simulink model "example"  (Simulink 8.5)
settings: Solver=ode15s  StartTime=0.0  StopTime=8*24*3600  RelTol=1e-3
undefined symbols (not defined in the file or in its folder): B, U, x0
settings Model: Creator=M.Sparnaaij  LastModifiedBy=Martijn  ExtModeTrigMode=oneshot  ExtModeArmWhenConnect=off
settings DataIOCC: LimitDataPoints=off  SignalLoggingName=sigsOut
settings OptimizationCC: BooleanDataType=off
settings DebuggingCC: SaveWithParameterizedLinksMsg=none  SignalResolutionControl=TryResolveAllWithWarning  MultiTaskDSMMsg=warning  MultiTaskCondExecSysMsg=none  FcnCallInpInsideContextMsg=EnableAllAsWarning  StrictBusMsg=None
settings HardwareCC: TargetUnknown=on

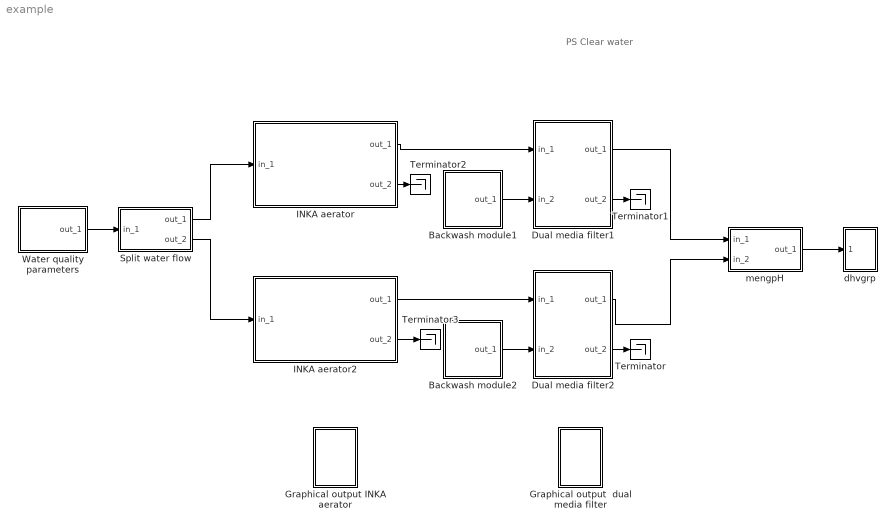
== system example ==
  note: PS Clear water
  Backwash module1 : Subsystem  Description=During a simulation the filter can be backwashed with the backwash module, so a number of successive filterruns can be simulated.
      mask init:
      | filenaam='./StimelaData/Backwash module1.mat';
      | 
      | [Pn,Fn,Fext]=Fileprop(filenaam);
      | 
      | errstr = st_UniqName(filenaam,'filenaam=''','SubSystem','OpenFcn');
      | if errstr, error([errstr 'The filename "' filenaam '" is already in use. Choose a different filename.']), end
      | 
      | P = bacwa1_p(filenaam);
      | [B,x0,U]=bacwa1_i(filenaam);
      settings: OpenFcn=|
      | filenaam='./StimelaData/Backwash module1.mat';
      | st_ParameterInput('init',gcb,filenaam,'bacwa1');
      mask Display:
      | plot(0,0,100,100,[80,80,20,20],[80,20,20,80],[40,42,38,40,40],[70,67,67,70,30],[60,62,58,60,60],[70,67,67,70,30]);
      | disp('')
      | text(50,50,'bacwa1', 'horizontalAlignment', 'center', 'verticalAlignment', 'middle');
      | text(50,0,Fn, 'horizontalAlignment', 'center', 'verticalAlignment', 'base');
  Backwash module2 : Subsystem  Description=During a simulation the filter can be backwashed with the backwash module, so a number of successive filterruns can be simulated.
      mask init:
      | filenaam='./StimelaData/Backwash module2.mat';
      | 
      | [Pn,Fn,Fext]=Fileprop(filenaam);
      | 
      | errstr = st_UniqName(filenaam,'filenaam=''','SubSystem','OpenFcn');
      | if errstr, error([errstr 'The filename "' filenaam '" is already in use. Choose a different filename.']), end
      | 
      | P = bacwa1_p(filenaam);
      | [B,x0,U]=bacwa1_i(filenaam);
      settings: OpenFcn=|
      | filenaam='./StimelaData/Backwash module2.mat';
      | st_ParameterInput('init',gcb,filenaam,'bacwa1');
      mask Display:
      | plot(0,0,100,100,[80,80,20,20],[80,20,20,80],[40,42,38,40,40],[70,67,67,70,30],[60,62,58,60,60],[70,67,67,70,30]);
      | disp('')
      | text(50,50,'bacwa1', 'horizontalAlignment', 'center', 'verticalAlignment', 'middle');
      | text(50,0,Fn, 'horizontalAlignment', 'center', 'verticalAlignment', 'base');
  Dual media filter1 : Subsystem  Description=This model calculates the removal of suspended solids with a dual media filter.
      mask init:
      | filenaam='./StimelaData/Dual_media_filter1.mat';
      | 
      | [Pn,Fn,Fext]=Fileprop(filenaam);
      | 
      | errstr = st_UniqName(filenaam,'filenaam=''','SubSystem','OpenFcn');
      | if errstr, error([errstr 'The filename "' filenaam '" is already in use. Choose a different filename.']), end
      | 
      | P = dubfil_p(filenaam);
      | [B,x0,U]=dubfil_i(filenaam);
      settings: OpenFcn=|
      | filenaam='./StimelaData/Dual_media_filter1.mat';
      | st_ParameterInput('init',gcb,filenaam,'dubfil');
      mask Display:
      | plot(0,0,100,100,[25.000000,25.000000,75.000000,75.000000,87.500000],[75.000000,25.000000,25.000000,30.000000,30.000000],[87.500000,75.000000,75.000000],[37.500000,37.500000,75.000000],[25.000000,75.000000],[65.000000,65.000000],[25.000000,75.000000],[42.500000,42.500000],[37.500000,42.500000],[52.500000,52.500000],[50.000000,55.000000],[52.500000,52.500000],[62.500000,67.500000],[52.500000,52.500000])
      | disp('')
      | text(50,50,'dubfil', 'horizontalAlignment', 'center', 'verticalAlignment', 'middle');
      | text(50,0,Fn, 'horizontalAlignment', 'center', 'verticalAlignment', 'base');
  Dual media filter2 : Subsystem  Description=This model calculates the removal of suspended solids with a dual media filter.
      mask init:
      | filenaam='./StimelaData/Dual_media_filter2.mat';
      | 
      | [Pn,Fn,Fext]=Fileprop(filenaam);
      | 
      | errstr = st_UniqName(filenaam,'filenaam=''','SubSystem','OpenFcn');
      | if errstr, error([errstr 'The filename "' filenaam '" is already in use. Choose a different filename.']), end
      | 
      | P = dubfil_p(filenaam);
      | [B,x0,U]=dubfil_i(filenaam);
      settings: OpenFcn=|
      | filenaam='./StimelaData/Dual_media_filter2.mat';
      | st_ParameterInput('init',gcb,filenaam,'dubfil');
      mask Display:
      | plot(0,0,100,100,[25.000000,25.000000,75.000000,75.000000,87.500000],[75.000000,25.000000,25.000000,30.000000,30.000000],[87.500000,75.000000,75.000000],[37.500000,37.500000,75.000000],[25.000000,75.000000],[65.000000,65.000000],[25.000000,75.000000],[42.500000,42.500000],[37.500000,42.500000],[52.500000,52.500000],[50.000000,55.000000],[52.500000,52.500000],[62.500000,67.500000],[52.500000,52.500000])
      | disp('')
      | text(50,50,'dubfil', 'horizontalAlignment', 'center', 'verticalAlignment', 'middle');
      | text(50,0,Fn, 'horizontalAlignment', 'center', 'verticalAlignment', 'base');
  Graphical output  dual media filter : Subsystem
      settings: OpenFcn=dubfil_g
      mask Display:
      | plot(0,0,100,100,[80,20,20],[20,20,80],[80,69,60,52,45,39,33,28,24,20],[65,65,64,61,57,52,45,37,30,20])
      | disp('');
      | text(100,100,'dubfil', 'horizontalAlignment', 'right', 'verticalAlignment', 'top');
  Graphical output INKA aerator : Subsystem
      settings: OpenFcn=plaatb_g
      mask Display:
      | plot(0,0,100,100,[80,20,20],[20,20,80],[80,69,60,52,45,39,33,28,24,20],[65,65,64,61,57,52,45,37,30,20])
      | disp('');
      | text(100,100,'plaatb', 'horizontalAlignment', 'right', 'verticalAlignment', 'top');
  INKA aerator : Subsystem  Description=This model calculates the aeration and degassifying with an INKA aerator. The influent carbon dioxide concentration is calculated on the basis of the bicarbonate concentration, the pH, the EGV and the water temperature, so these parameters must always be filled out in the 'Water quality parameters' block.
      mask init:
      | filenaam='./StimelaData/INKA_aerator1.mat';
      | 
      | [Pn,Fn,Fext]=Fileprop(filenaam);
      | 
      | errstr = st_UniqName(filenaam,'filenaam=''','SubSystem','OpenFcn');
      | if errstr, error([errstr 'The filename "' filenaam '" is already in use. Choose a different filename.']), end
      | 
      | P = plaatb_p(filenaam);
      | [B,x0,U]=plaatb_i(filenaam);
      settings: OpenFcn=|
      | filenaam='./StimelaData/INKA_aerator1.mat';
      | st_ParameterInput('init',gcb,filenaam,'plaatb');
      mask Display:
      | plot(0,0,100,100,[20,80,80,20,20],[70,70,20,20,70],[80,90,90,90,9,9,20],[20,20,30,40,40,60,60],[80,20],[50,50],[11,10,8,6],[60,65,68,70],[15,14,12,10,6],[60,64,67,69,70],[78,78],[40,50],[84,83,82,80],[40,45,48,50],[87,86,84,80],[40,45,48,50],[64,64,67,67],[80,77,77,70],[64,73,73,70,70],[80,80,77,77,70],[70,67],[77,77])
      | disp('')
      | text(50,50,'plaatb', 'horizontalAlignment', 'center', 'verticalAlignment', 'middle');
      | text(50,0,Fn, 'horizontalAlignment', 'center', 'verticalAlignment', 'base');
  INKA aerator2 : Subsystem  Description=This model calculates the aeration and degassifying with an INKA aerator. The influent carbon dioxide concentration is calculated on the basis of the bicarbonate concentration, the pH, the EGV and the water temperature, so these parameters must always be filled out in the 'Water quality parameters' block.
      mask init:
      | filenaam='./StimelaData/INKA_aerator2.mat';
      | 
      | [Pn,Fn,Fext]=Fileprop(filenaam);
      | 
      | errstr = st_UniqName(filenaam,'filenaam=''','SubSystem','OpenFcn');
      | if errstr, error([errstr 'The filename "' filenaam '" is already in use. Choose a different filename.']), end
      | 
      | P = plaatb_p(filenaam);
      | [B,x0,U]=plaatb_i(filenaam);
      settings: OpenFcn=|
      | filenaam='./StimelaData/INKA_aerator2.mat';
      | st_ParameterInput('init',gcb,filenaam,'plaatb');
      mask Display:
      | plot(0,0,100,100,[20,80,80,20,20],[70,70,20,20,70],[80,90,90,90,9,9,20],[20,20,30,40,40,60,60],[80,20],[50,50],[11,10,8,6],[60,65,68,70],[15,14,12,10,6],[60,64,67,69,70],[78,78],[40,50],[84,83,82,80],[40,45,48,50],[87,86,84,80],[40,45,48,50],[64,64,67,67],[80,77,77,70],[64,73,73,70,70],[80,80,77,77,70],[70,67],[77,77])
      | disp('')
      | text(50,50,'plaatb', 'horizontalAlignment', 'center', 'verticalAlignment', 'middle');
      | text(50,0,Fn, 'horizontalAlignment', 'center', 'verticalAlignment', 'base');
  Split water flow : Subsystem  Description=splits
      mask init:
      | filenaam='./StimelaData/splits_p.mat';
      | 
      | [Pn,Fn,Fext]=Fileprop(filenaam);
      | 
      | errstr = st_UniqName(filenaam,'filenaam=''','SubSystem','OpenFcn');
      | if errstr, error([errstr 'The filename "' filenaam '" is already in use. Choose a different filename.']), end
      | 
      | P = splits_p(filenaam);
      | [B,x0,U]=splits_i(filenaam);
      settings: OpenFcn=|
      | filenaam='./StimelaData/splits_p.mat';
      | st_ParameterInput('init',gcb,filenaam,'splits');
      mask Display:
      | plot(0,0,100,100,[0 20],[50 50],[0 20],[55 55],[80 100],[80 80],[80 100],[85 85],[80 100],[ 20 20],[80 100],[ 15 15],[20 80 80 20 20],[10 10 90  90 10]);
      | disp('')
      | text(50,50,'splits', 'horizontalAlignment', 'center', 'verticalAlignment', 'middle');
      | text(50,0,Fn, 'horizontalAlignment', 'center', 'verticalAlignment', 'base');
  Terminator{,1..3} (4 alike) : Terminator
  Water quality parameters : Subsystem  Description=The water flow and the water quality data must be filled out in the 'Water quality parameters' block. Each project must start with a 'Water quality parameters' block.
      mask init:
      | filenaam='./StimelaData/Water_qual_param.mat';
      | 
      | [Pn,Fn,Fext]=Fileprop(filenaam);
      | 
      | errstr = st_UniqName(filenaam,'filenaam=''','SubSystem','OpenFcn');
      | if errstr, error([errstr 'The filename "' filenaam '" is already in use. Choose a different filename.']), end
      | 
      | P = invruw_p(filenaam);
      | [B,x0,U]=invruw_i(filenaam);
      settings: OpenFcn=|
      | filenaam='./StimelaData/Water_qual_param.mat';
      | st_ParameterInput('init',gcb,filenaam,'invruw');
      mask Display:
      | plot(0,0,100,100,[80 100],[ 50 50],[80 100],[ 55 55],[20 80 80 20 20],[10 10 90  90 10]);
      | disp('')
      | text(50,50,'invruw', 'horizontalAlignment', 'center', 'verticalAlignment', 'middle');
      | text(50,0,Fn, 'horizontalAlignment', 'center', 'verticalAlignment', 'base');
  dhvgrp : Subsystem  Description=dhvgrp
      mask init:
      | filenaam='./StimelaData/OnLineGraph.mat';
      | 
      | [Pn,Fn,Fext]=Fileprop(filenaam);
      | 
      | errstr = st_UniqName(filenaam,'filenaam=''','SubSystem','OpenFcn');
      | if errstr, error([errstr 'The filename "' filenaam '" is already in use. Choose a different filename.']), end
      | 
      | P = dhvgrp_p(filenaam);
      | [B,x0,U]=dhvgrp_i(filenaam);
      settings: OpenFcn=|
      | filenaam='./StimelaData/OnLineGraph.mat';
      | st_ParameterInput('init',gcb,filenaam,'dhvgrp');
      mask Display:
      | plot(0,0,100,100,[90,10,10,10,90,90,10],[65,65,90,40,40,90,90],[90,78,69,54,40,31,25,10],[77,60,48,46,56,75,81,84])
      | disp('')
  mengpH : Subsystem  Description=mengpH
      mask init:
      | filenaam='./StimelaData/mengpH_p.mat';
      | 
      | [Pn,Fn,Fext]=Fileprop(filenaam);
      | 
      | errstr = st_UniqName(filenaam,'filenaam=''','SubSystem','OpenFcn');
      | if errstr, error([errstr 'The filename "' filenaam '" is already in use. Choose a different filename.']), end
      | 
      | P = mengpH_p(filenaam);
      | [B,x0,U]=mengpH_i(filenaam);
      | V = st_Varia;
      settings: OpenFcn=|
      | filenaam='./StimelaData/mengpH_p.mat';
      | st_ParameterInput('init',gcb,filenaam,'mengpH');
      mask Display:
      | plot(0,0,100,100,[0 20],[85 85],[0 20],[80 80],[0 20],[20 20],[0 20],[15 15],[80 100],[ 50 50],[80 100],[ 55 55],[20 80 80 20 20],[10 10 90  90 10]);
      | disp('')
      | text(50,50,'mengpH', 'horizontalAlignment', 'center', 'verticalAlignment', 'middle');
      | text(50,0,Fn, 'horizontalAlignment', 'center', 'verticalAlignment', 'base');
  wires:
  Split water flow/2(out_2) -> INKA aerator2/1(in_1)
  Split water flow/1(out_1) -> INKA aerator/1(in_1)
  Water quality parameters/1(out_1) -> Split water flow/1(in_1)
  INKA aerator/1(out_1) -> Dual media filter1/1(in_1)
  INKA aerator2/1(out_1) -> Dual media filter2/1(in_1)
  Dual media filter1/1(out_1) -> mengpH/1(in_1)
  Dual media filter2/1(out_1) -> mengpH/2(in_2)
  Backwash module2/1(out_1) -> Dual media filter2/2(in_2)
  Dual media filter2/2(out_2) -> Terminator/1
  Dual media filter1/2(out_2) -> Terminator1/1
  INKA aerator/2(out_2) -> Terminator2/1
  INKA aerator2/2(out_2) -> Terminator3/1
  Backwash module1/1(out_1) -> Dual media filter1/2(in_2)
  mengpH/1(out_1) -> dhvgrp/1(in_1)

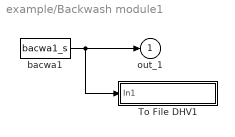
== system example/Backwash module1 ==
  To File DHV1 : Subsystem  mask(To File DHV){naam=[filenaam(1:length(filenaam)-4) '_out.sti']}
      mask prompts: naam "Naam van bestand"
      mask init:
      | set_param([gcb '/To File'],'Filename',naam);
      mask Display: disp(naam)
  bacwa1 : S-Function  FunctionName=bacwa1_s  Parameters=B,x0,U,P
  out_1 : Outport  InitialOutput=0
  wires:
  bacwa1/1 -> out_1/1, To File DHV1/1(In1)

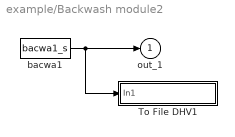
== system example/Backwash module2 ==
  To File DHV1 : Subsystem  mask(To File DHV){naam=[filenaam(1:length(filenaam)-4) '_out.sti']}
      mask prompts: naam "Naam van bestand"
      mask init:
      | set_param([gcb '/To File'],'Filename',naam);
      mask Display: disp(naam)
  bacwa1 : S-Function  FunctionName=bacwa1_s  Parameters=B,x0,U,P
  out_1 : Outport  InitialOutput=0
  wires:
  bacwa1/1 -> out_1/1, To File DHV1/1(In1)

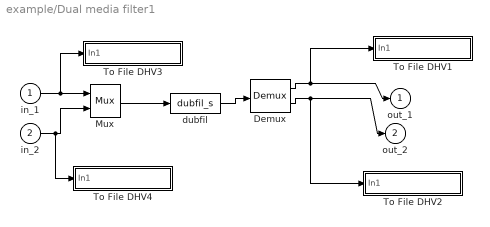
== system example/Dual media filter1 ==
  in_1 : Inport
  in_2 : Inport  Port=2
  Demux : Demux  Outputs=[U.Number B.Measurements]
  Mux : Mux  Inputs=[U.Number B.Setpoints]
  To File DHV1 : Subsystem  mask(To File DHV){naam=[filenaam(1:length(filenaam)-4) '_out.sti']}
      mask prompts: naam "Naam van bestand"
      mask init:
      | set_param([gcb '/To File'],'Filename',naam);
      mask Display: disp(naam)
  To File DHV2 : Subsystem  mask(To File DHV){naam=[filenaam(1:length(filenaam)-4) '_EM.sti']}
      mask prompts: naam "Naam van bestand"
      mask init:
      | set_param([gcb '/To File'],'Filename',naam);
      mask Display: disp(naam)
  To File DHV3 : Subsystem  mask(To File DHV){naam=[filenaam(1:length(filenaam)-4) '_in.sti']}
      mask prompts: naam "Naam van bestand"
      mask init:
      | set_param([gcb '/To File'],'Filename',naam);
      mask Display: disp(naam)
  To File DHV4 : Subsystem  mask(To File DHV){naam=[filenaam(1:length(filenaam)-4) '_ES.sti']}
      mask prompts: naam "Naam van bestand"
      mask init:
      | set_param([gcb '/To File'],'Filename',naam);
      mask Display: disp(naam)
  dubfil : S-Function  FunctionName=dubfil_s  Parameters=B,x0,U,P
  out_1 : Outport  InitialOutput=0
  out_2 : Outport  Port=2  InitialOutput=0
  wires:
  Demux/2 -> out_2/1, To File DHV2/1(In1)
  Demux/1 -> out_1/1, To File DHV1/1(In1)
  dubfil/1 -> Demux/1
  in_1/1 -> Mux/1, To File DHV3/1(In1)
  Mux/1 -> dubfil/1
  in_2/1 -> Mux/2, To File DHV4/1(In1)

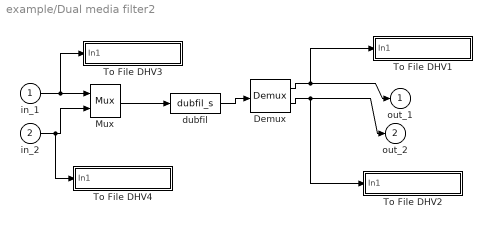
== system example/Dual media filter2 ==
  in_1 : Inport
  in_2 : Inport  Port=2
  Demux : Demux  Outputs=[U.Number B.Measurements]
  Mux : Mux  Inputs=[U.Number B.Setpoints]
  To File DHV1 : Subsystem  mask(To File DHV){naam=[filenaam(1:length(filenaam)-4) '_out.sti']}
      mask prompts: naam "Naam van bestand"
      mask init:
      | set_param([gcb '/To File'],'Filename',naam);
      mask Display: disp(naam)
  To File DHV2 : Subsystem  mask(To File DHV){naam=[filenaam(1:length(filenaam)-4) '_EM.sti']}
      mask prompts: naam "Naam van bestand"
      mask init:
      | set_param([gcb '/To File'],'Filename',naam);
      mask Display: disp(naam)
  To File DHV3 : Subsystem  mask(To File DHV){naam=[filenaam(1:length(filenaam)-4) '_in.sti']}
      mask prompts: naam "Naam van bestand"
      mask init:
      | set_param([gcb '/To File'],'Filename',naam);
      mask Display: disp(naam)
  To File DHV4 : Subsystem  mask(To File DHV){naam=[filenaam(1:length(filenaam)-4) '_ES.sti']}
      mask prompts: naam "Naam van bestand"
      mask init:
      | set_param([gcb '/To File'],'Filename',naam);
      mask Display: disp(naam)
  dubfil : S-Function  FunctionName=dubfil_s  Parameters=B,x0,U,P
  out_1 : Outport  InitialOutput=0
  out_2 : Outport  Port=2  InitialOutput=0
  wires:
  Demux/2 -> out_2/1, To File DHV2/1(In1)
  Demux/1 -> out_1/1, To File DHV1/1(In1)
  dubfil/1 -> Demux/1
  in_1/1 -> Mux/1, To File DHV3/1(In1)
  Mux/1 -> dubfil/1
  in_2/1 -> Mux/2, To File DHV4/1(In1)

== system example/Graphical output  dual media filter ==
  note: plotten

== system example/Graphical output INKA aerator ==
  note: plotten

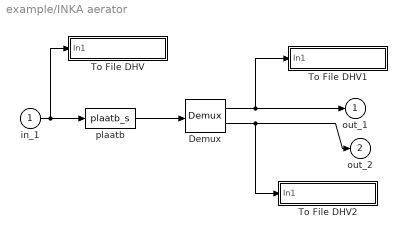
== system example/INKA aerator ==
  in_1 : Inport
  Demux : Demux  Outputs=[U.Number B.Measurements]
  To File DHV : Subsystem  mask(To File DHV){naam=[filenaam(1:length(filenaam)-4) '_in.sti']}
      mask prompts: naam "Naam van bestand"
      mask init:
      | set_param([gcb '/To File'],'Filename',naam);
      mask Display: disp(naam)
  To File DHV1 : Subsystem  mask(To File DHV){naam=[filenaam(1:length(filenaam)-4) '_out.sti']}
      mask prompts: naam "Naam van bestand"
      mask init:
      | set_param([gcb '/To File'],'Filename',naam);
      mask Display: disp(naam)
  To File DHV2 : Subsystem  mask(To File DHV){naam=[filenaam(1:length(filenaam)-4) '_EM.sti']}
      mask prompts: naam "Naam van bestand"
      mask init:
      | set_param([gcb '/To File'],'Filename',naam);
      mask Display: disp(naam)
  plaatb : S-Function  FunctionName=plaatb_s  Parameters=B,x0,U,P
  out_1 : Outport  InitialOutput=0
  out_2 : Outport  Port=2  InitialOutput=0
  wires:
  plaatb/1 -> Demux/1
  Demux/1 -> out_1/1, To File DHV1/1(In1)
  Demux/2 -> out_2/1, To File DHV2/1(In1)
  in_1/1 -> plaatb/1, To File DHV/1(In1)

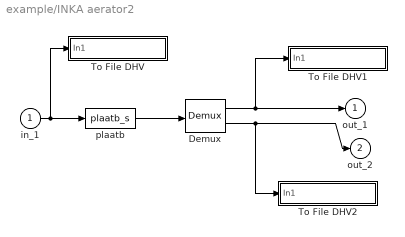
== system example/INKA aerator2 ==
  in_1 : Inport
  Demux : Demux  Outputs=[U.Number B.Measurements]
  To File DHV : Subsystem  mask(To File DHV){naam=[filenaam(1:length(filenaam)-4) '_in.sti']}
      mask prompts: naam "Naam van bestand"
      mask init:
      | set_param([gcb '/To File'],'Filename',naam);
      mask Display: disp(naam)
  To File DHV1 : Subsystem  mask(To File DHV){naam=[filenaam(1:length(filenaam)-4) '_out.sti']}
      mask prompts: naam "Naam van bestand"
      mask init:
      | set_param([gcb '/To File'],'Filename',naam);
      mask Display: disp(naam)
  To File DHV2 : Subsystem  mask(To File DHV){naam=[filenaam(1:length(filenaam)-4) '_EM.sti']}
      mask prompts: naam "Naam van bestand"
      mask init:
      | set_param([gcb '/To File'],'Filename',naam);
      mask Display: disp(naam)
  plaatb : S-Function  FunctionName=plaatb_s  Parameters=B,x0,U,P
  out_1 : Outport  InitialOutput=0
  out_2 : Outport  Port=2  InitialOutput=0
  wires:
  plaatb/1 -> Demux/1
  Demux/1 -> out_1/1, To File DHV1/1(In1)
  Demux/2 -> out_2/1, To File DHV2/1(In1)
  in_1/1 -> plaatb/1, To File DHV/1(In1)

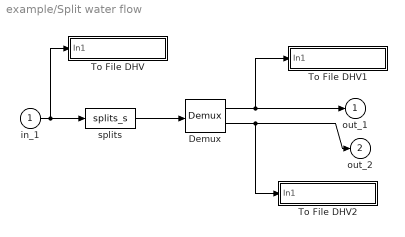
== system example/Split water flow ==
  in_1 : Inport
  Demux : Demux  Outputs=[U.Number B.Measurements]
  To File DHV : Subsystem  mask(To File DHV){naam=[filenaam(1:length(filenaam)-4) '_in.sti']}
      mask prompts: naam "Naam van bestand"
      mask init:
      | set_param([gcb '/To File'],'Filename',naam);
      mask Display: disp(naam)
  To File DHV1 : Subsystem  mask(To File DHV){naam=[filenaam(1:length(filenaam)-4) '_out.sti']}
      mask prompts: naam "Naam van bestand"
      mask init:
      | set_param([gcb '/To File'],'Filename',naam);
      mask Display: disp(naam)
  To File DHV2 : Subsystem  mask(To File DHV){naam=[filenaam(1:length(filenaam)-4) '_EM.sti']}
      mask prompts: naam "Naam van bestand"
      mask init:
      | set_param([gcb '/To File'],'Filename',naam);
      mask Display: disp(naam)
  splits : S-Function  FunctionName=splits_s  Parameters=B,x0,U,P
  out_1 : Outport  InitialOutput=0
  out_2 : Outport  Port=2  InitialOutput=0
  wires:
  splits/1 -> Demux/1
  Demux/1 -> out_1/1, To File DHV1/1(In1)
  Demux/2 -> out_2/1, To File DHV2/1(In1)
  in_1/1 -> splits/1, To File DHV/1(In1)

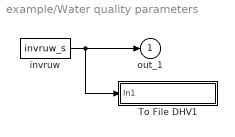
== system example/Water quality parameters ==
  To File DHV1 : Subsystem  mask(To File DHV){naam=[filenaam(1:length(filenaam)-4) '_out.sti']}
      mask prompts: naam "Naam van bestand"
      mask init:
      | set_param([gcb '/To File'],'Filename',naam);
      mask Display: disp(naam)
  invruw : S-Function  FunctionName=invruw_s  Parameters=B,x0,U,P
  out_1 : Outport  InitialOutput=0
  wires:
  invruw/1 -> out_1/1, To File DHV1/1(In1)

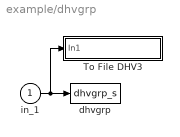
== system example/dhvgrp ==
  in_1 : Inport
  To File DHV3 : Subsystem  mask(To File DHV){naam=[filenaam(1:length(filenaam)-4) '_in.sti']}
      mask prompts: naam "Naam van bestand"
      mask init:
      | set_param([gcb '/To File'],'Filename',naam);
      mask Display: disp(naam)
  dhvgrp : S-Function  FunctionName=dhvgrp_s  Parameters=B,x0,U,P
  wires:
  in_1/1 -> To File DHV3/1(In1), dhvgrp/1

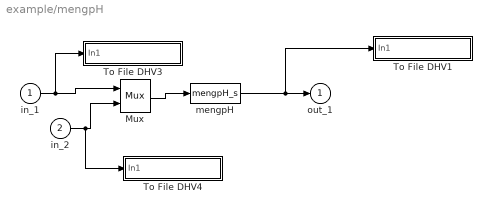
== system example/mengpH ==
  in_1 : Inport
  in_2 : Inport  Port=2
  Mux : Mux  Inputs=[U.Number B.Setpoints]
  To File DHV1 : Subsystem  mask(To File DHV){naam=[filenaam(1:length(filenaam)-4) '_out.sti']}
      mask prompts: naam "Naam van bestand"
      mask init:
      | set_param([gcb '/To File'],'Filename',naam);
      mask Display: disp(naam)
  To File DHV3 : Subsystem  mask(To File DHV){naam=[filenaam(1:length(filenaam)-4) '_in.sti']}
      mask prompts: naam "Naam van bestand"
      mask init:
      | set_param([gcb '/To File'],'Filename',naam);
      mask Display: disp(naam)
  To File DHV4 : Subsystem  mask(To File DHV){naam=[filenaam(1:length(filenaam)-4) '_ES.sti']}
      mask prompts: naam "Naam van bestand"
      mask init:
      | set_param([gcb '/To File'],'Filename',naam);
      mask Display: disp(naam)
  mengpH : S-Function  FunctionName=mengpH_s  Parameters=B,x0,U,P
  out_1 : Outport  InitialOutput=0
  wires:
  mengpH/1 -> out_1/1, To File DHV1/1(In1)
  Mux/1 -> mengpH/1
  in_1/1 -> Mux/1, To File DHV3/1(In1)
  in_2/1 -> Mux/2, To File DHV4/1(In1)

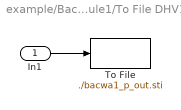
== system example/Backwash module1/To File DHV1 ==
  In1 : Inport
  To File : ToFile  Filename=./bacwa1_p_out.sti  MatrixName=bacwa1out
  wires:
  In1/1 -> To File/1

== system example/Backwash module2/To File DHV1 ==
  In1 : Inport
  To File : ToFile  Filename=./bacwa1_p_out.sti  MatrixName=bacwa1out
  wires:
  In1/1 -> To File/1

== system example/Dual media filter1/To File DHV1 ==
  In1 : Inport
  To File : ToFile  Filename=./dubfil_p_out.sti  MatrixName=dubfilout
  wires:
  In1/1 -> To File/1

== system example/Dual media filter1/To File DHV2 ==
  In1 : Inport
  To File : ToFile  Filename=./dubfil_p_EM.sti  MatrixName=dubfilEM
  wires:
  In1/1 -> To File/1

== system example/Dual media filter1/To File DHV3 ==
  In1 : Inport
  To File : ToFile  Filename=./dubfil_p_in.sti  MatrixName=dubfilin
  wires:
  In1/1 -> To File/1

== system example/Dual media filter1/To File DHV4 ==
  In1 : Inport
  To File : ToFile  Filename=./dubfil_p_ES.sti  MatrixName=dubfilES
  wires:
  In1/1 -> To File/1

== system example/Dual media filter2/To File DHV1 ==
  In1 : Inport
  To File : ToFile  Filename=./dubfil_p_out.sti  MatrixName=dubfilout
  wires:
  In1/1 -> To File/1

== system example/Dual media filter2/To File DHV2 ==
  In1 : Inport
  To File : ToFile  Filename=./dubfil_p_EM.sti  MatrixName=dubfilEM
  wires:
  In1/1 -> To File/1

== system example/Dual media filter2/To File DHV3 ==
  In1 : Inport
  To File : ToFile  Filename=./dubfil_p_in.sti  MatrixName=dubfilin
  wires:
  In1/1 -> To File/1

== system example/Dual media filter2/To File DHV4 ==
  In1 : Inport
  To File : ToFile  Filename=./dubfil_p_ES.sti  MatrixName=dubfilES
  wires:
  In1/1 -> To File/1

== system example/INKA aerator/To File DHV ==
  In1 : Inport
  To File : ToFile  Filename=./plaatb_p_in.sti  MatrixName=plaatbin
  wires:
  In1/1 -> To File/1

== system example/INKA aerator/To File DHV1 ==
  In1 : Inport
  To File : ToFile  Filename=./plaatb_p_out.sti  MatrixName=plaatbout
  wires:
  In1/1 -> To File/1

== system example/INKA aerator/To File DHV2 ==
  In1 : Inport
  To File : ToFile  Filename=./plaatb_p_EM.sti  MatrixName=plaatbEM
  wires:
  In1/1 -> To File/1

== system example/INKA aerator2/To File DHV ==
  In1 : Inport
  To File : ToFile  Filename=./plaatb_p_in.sti  MatrixName=plaatbin
  wires:
  In1/1 -> To File/1

== system example/INKA aerator2/To File DHV1 ==
  In1 : Inport
  To File : ToFile  Filename=./plaatb_p_out.sti  MatrixName=plaatbout
  wires:
  In1/1 -> To File/1

== system example/INKA aerator2/To File DHV2 ==
  In1 : Inport
  To File : ToFile  Filename=./plaatb_p_EM.sti  MatrixName=plaatbEM
  wires:
  In1/1 -> To File/1

== system example/Split water flow/To File DHV ==
  In1 : Inport
  To File : ToFile  Filename=./splits_p_in.sti  MatrixName=splitsin
  wires:
  In1/1 -> To File/1

== system example/Split water flow/To File DHV1 ==
  In1 : Inport
  To File : ToFile  Filename=./splits_p_out.sti  MatrixName=splitsout
  wires:
  In1/1 -> To File/1

== system example/Split water flow/To File DHV2 ==
  In1 : Inport
  To File : ToFile  Filename=./splits_p_EM.sti  MatrixName=splitsEM
  wires:
  In1/1 -> To File/1

== system example/Water quality parameters/To File DHV1 ==
  In1 : Inport
  To File : ToFile  Filename=./invruw_p_out.sti  MatrixName=invruwout
  wires:
  In1/1 -> To File/1

== system example/dhvgrp/To File DHV3 ==
  In1 : Inport
  To File : ToFile  Filename=./dhvgrp_p_in.sti  MatrixName=dhvgrpin
  wires:
  In1/1 -> To File/1

== system example/mengpH/To File DHV1 ==
  In1 : Inport
  To File : ToFile  Filename=./mengpH_p_out.sti  MatrixName=mengpHout
  wires:
  In1/1 -> To File/1

== system example/mengpH/To File DHV3 ==
  In1 : Inport
  To File : ToFile  Filename=./mengpH_p_in.sti  MatrixName=mengpHin
  wires:
  In1/1 -> To File/1

== system example/mengpH/To File DHV4 ==
  In1 : Inport
  To File : ToFile  Filename=./mengpH_p_ES.sti  MatrixName=mengpHES
  wires:
  In1/1 -> To File/1
